simulink library "motohawk_engine_motoshare_lib"  (Simulink 6.3)
undefined symbols (not defined in the file or in its folder): cast_val, IndPowerMax, lookup_group, motohawk_tex, motohawk_vardec_config_group, motohawk_vardec_path, SampleTime, SteadyStateECT, txtTitle, WarmUpTimeConst
libraries: MotoHawk_lib x211, motohawk_control_primitives_lib x20, motohawk_annotations_lib x7, motohawk_engine_lib x5, AutoDoc_lib x4, motohawk_control_primitives_lib_new x3, motohawk_control_primitives_motoshare_lib x2
(part 5 of 7)

== system motohawk_engine_motoshare_lib/PWM Characterization ==
  note: The outputs of this block are designed to be
      | directly connected to a MotoHawk PWM block.
  EngUnits : Inport
  Convert to integer 0.01Hz resolution : Gain  Gain=100  SaturateOnIntegerOverflow=on
  Convert to integer 14-bit PWM resolution : Gain  Gain=40.95  SaturateOnIntegerOverflow=on
  Data Type Conversion1 : DataTypeConversion  SaturateOnIntegerOverflow=on  RndMeth=Zero
  Data Type Conversion2 : DataTypeConversion  OutDataTypeMode=uint32  SaturateOnIntegerOverflow=on  RndMeth=Zero
  Data Type Conversion3 : DataTypeConversion  OutDataTypeMode=int16  SaturateOnIntegerOverflow=on  RndMeth=Zero
  Product : Product  SaturateOnIntegerOverflow=on  InputSameDT=on
  Saturation : motohawk_control_primitives_lib/Saturation
  Sum : Sum  Inputs=|++  SaturateOnIntegerOverflow=on
  motohawk_calibration : MotoHawk_lib/Calibration & Probing Blocks/motohawk_calibration  nam=[prefix 'Gain']  val=1  storage=Calibration  show_more=on  name_source=Use Parameter  data_type=double  read_level=1  write_level=1  ovr_cals=on  view_as=Number  enum_struct={'Disabled', 'Enabled'}  vector_style=Wide Row  use_help_units=on  help='Scaling from engineering units to PWM duty cycle'  units=['%/' units]  use_header_enum=off  row_header_enum={}  col_header_enum={}  use_min_max=off  min_val=-inf  max_val=inf  use_precision=off  precision=''  gain=1  offset=0  exp=1  use_mototune_group=on  mototune_group=[group ' | ' nam ' Config']
  motohawk_calibration1 : MotoHawk_lib/Calibration & Probing Blocks/motohawk_calibration  nam=[prefix 'Offset']  val=0  storage=Calibration  show_more=on  name_source=Use Parameter  data_type=double  read_level=1  write_level=1  ovr_cals=on  view_as=Number  enum_struct={'Disabled', 'Enabled'}  vector_style=Wide Row  use_help_units=on  help='Offset from engineering units to PWM duty cycle'  units='%'  use_header_enum=off  row_header_enum={}  col_header_enum={}  use_min_max=off  min_val=-inf  max_val=inf  use_precision=off  precision=''  gain=1  offset=0  exp=1  use_mototune_group=on  mototune_group=[group ' | ' nam ' Config']
  motohawk_calibration2 : MotoHawk_lib/Calibration & Probing Blocks/motohawk_calibration  nam=[prefix 'MinLimit']  val=0  storage=Calibration  show_more=on  name_source=Use Parameter  data_type=double  read_level=1  write_level=1  ovr_cals=on  view_as=Number  enum_struct={'Disabled', 'Enabled'}  vector_style=Wide Row  use_help_units=on  help='Minimum limit of PWM signal.'  units='%'  use_header_enum=off  row_header_enum={}  col_header_enum={}  use_min_max=off  min_val=-inf  max_val=inf  use_precision=off  precision=''  gain=1  offset=0  exp=1  use_mototune_group=on  mototune_group=[group ' | ' nam ' Config']
  motohawk_calibration3 : MotoHawk_lib/Calibration & Probing Blocks/motohawk_calibration  nam=[prefix 'MaxLimit']  val=100  storage=Calibration  show_more=on  name_source=Use Parameter  data_type=double  read_level=1  write_level=1  ovr_cals=on  view_as=Number  enum_struct={'Disabled', 'Enabled'}  vector_style=Wide Row  use_help_units=on  help='Maximum limit of PWM signal.'  units='%'  use_header_enum=off  row_header_enum={}  col_header_enum={}  use_min_max=off  min_val=-inf  max_val=inf  use_precision=off  precision=''  gain=1  offset=0  exp=1  use_mototune_group=on  mototune_group=[group ' | ' nam ' Config']
  motohawk_calibration4 : MotoHawk_lib/Calibration & Probing Blocks/motohawk_calibration  nam=[prefix 'Frequency']  val=100  storage=Calibration  show_more=on  name_source=Use Parameter  data_type=double  read_level=1  write_level=1  ovr_cals=on  view_as=Number  enum_struct={'Disabled', 'Enabled'}  vector_style=Wide Row  use_help_units=on  help='Frequency of PWM output'  units='Hz'  use_header_enum=off  row_header_enum={}  col_header_enum={}  use_min_max=off  min_val=-inf  max_val=inf  use_precision=off  precision=''  gain=1  offset=0  exp=1  use_mototune_group=on  mototune_group=[group ' | ' nam ' Config']
  motohawk_override_abs2 : MotoHawk_lib/Calibration & Probing Blocks/motohawk_override_abs  parent_name=nam  show_more=on  name_source=Use Parameter  parent_read_level=1  parent_override_level=1  view_as=Number  enum_struct={'Disabled', 'Enabled'}  use_help_units=on  parent_help='Override result of linear sensor characterization, in engineering units'  parent_units=units  use_min_max=on  parent_min=-inf  parent_max=inf  use_precision=off  parent_precision=''  parent_gain=1  parent_offset=0  parent_exp=1  use_mototune_group=on  parent_group=group
  motohawk_probe2 : MotoHawk_lib/Calibration & Probing Blocks/motohawk_probe  nam=[prefix 'DutyCycle']  show_more=on  name_source=Use Parameter  read_level=1  view_as=Number  enum_struct={'Disabled', 'Enabled'}  vector_style=Wide Row  use_help_units=on  help='Actual duty cycle of actuator'  units='%'  use_header_enum=off  row_header_enum={}  col_header_enum={}  use_precision=off  precision=''  gain=1  offset=0  exp=1  use_mototune_group=on  mototune_group=group
  DutyCycle : Outport
  Frequency : Outport  Port=2
  wires:
  Data Type Conversion2/1 -> Frequency/1
  Convert to integer 0.01Hz resolution/1 -> Data Type Conversion2/1
  motohawk_calibration4/1 -> Convert to integer 0.01Hz resolution/1
  Data Type Conversion1/1 -> Product/1
  motohawk_override_abs2/1 -> Data Type Conversion1/1
  EngUnits/1 -> motohawk_override_abs2/1
  Product/1 -> Sum/1
  motohawk_calibration1/1 -> Sum/2
  motohawk_calibration/1 -> Product/2
  Data Type Conversion3/1 -> DutyCycle/1
  Convert to integer 14-bit PWM resolution/1 -> Data Type Conversion3/1
  Sum/1 -> Saturation/1
  Saturation/1 -> Convert to integer 14-bit PWM resolution/1, motohawk_probe2/1
  motohawk_calibration2/1 -> Saturation/2
  motohawk_calibration3/1 -> Saturation/3

== system motohawk_engine_motoshare_lib/Spark Coil Characterization ==
  SparkEnergy [mJ] : Inport
  SysVolt09Idx : Inport  Port=2
  Constant : Constant  Value=1000
  Constant1 : Constant  Value=0
  Only Enable Spark when Energy is Above Zero : RelationalOperator  Operator=>  ZeroCross=off  InputSameDT=on
  Product : Product  Inputs=*/  SaturateOnIntegerOverflow=on
  Sum : Sum  Inputs=|++  SaturateOnIntegerOverflow=on
  motohawk_calibration : MotoHawk_lib/Calibration & Probing Blocks/motohawk_calibration  nam='CoilDrvrDlyTime'  val=0  storage=Calibration  show_more=on  name_source=Use Parameter  data_type=Inherit from 'Default Value'  read_level=1  write_level=1  ovr_cals=on  view_as=Number  enum_struct={'Disabled', 'Enabled'}  vector_style=Wide Row  use_help_units=on  help='Spark Coil Driver Delay Time'  units='us'  use_header_enum=off  row_header_enum={}  col_header_enum={}  use_min_max=off  min_val=-inf  max_val=inf  use_precision=off  precision=''  gain=1  offset=0  exp=1  use_mototune_group=on  mototune_group=[group ' | Coil Config']
  motohawk_interpolation_2d : MotoHawk_lib/Lookup Tables/motohawk_interpolation_2d  nam='CoilDwell'  table_data=ones(9)  show_more=on  data_type=Inherit from 'Table Data'  storage=NonAdaptive  read_level=1  write_level=1  ovr_cals=on  use_help=on  help='Spark dwell time'  units='ms'  use_min_max=off  min_val=-inf  max_val=inf  use_precision=off  precision=''  gain=1  offset=0  exp=1  use_links=on  row_prelookup_block=''  col_prelookup_block=''  output_name='CoilDwell'  use_mototune_group=on  mototune_group=group
  motohawk_prelookup1 : MotoHawk_lib/Lookup Tables/motohawk_prelookup  nam='SpkEnergy09'  breakpoint_data=ones(1,9)  show_more=on  data_type=Inherit from 'Table Data'  storage=Constant  read_level=1  write_level=1  ovr_cals=on  use_help=on  help='Prelookup for Spark Energy'  units='mJ'  use_min_max=off  min_val=-inf  max_val=inf  use_precision=off  precision=''  gain=1  offset=0  exp=1  use_links=on  input_name='SparkEnergy'  use_mototune_group=on  mototune_group='Indexes'
  motohawk_probe : MotoHawk_lib/Calibration & Probing Blocks/motohawk_probe  nam='CoilDwell'  show_more=on  name_source=Use Parameter  read_level=1  view_as=Number  enum_struct={'Disabled', 'Enabled'}  vector_style=Wide Row  use_help_units=on  help='Total electrical spark dwell time'  units='ms'  use_header_enum=off  row_header_enum={}  col_header_enum={}  use_precision=off  precision=''  gain=1  offset=0  exp=1  use_mototune_group=on  mototune_group=group
  motohawk_probe1 : MotoHawk_lib/Calibration & Probing Blocks/motohawk_probe  nam='SparkEnergy'  show_more=on  name_source=Use Parameter  read_level=1  view_as=Number  enum_struct={'Disabled', 'Enabled'}  vector_style=Wide Row  use_help_units=on  help='Commanded spark energy, before conversion to dwell time'  units='mJ'  use_header_enum=off  row_header_enum={}  col_header_enum={}  use_precision=off  precision=''  gain=1  offset=0  exp=1  use_mototune_group=on  mototune_group=group
  SparkDwell [ms] : Outport
  SparkEnable [bool] : Outport  Port=2
  wires:
  Constant1/1 -> Only Enable Spark when Energy is Above Zero/2
  Only Enable Spark when Energy is Above Zero/1 -> SparkEnable [bool]/1
  Constant/1 -> Product/2
  Product/1 -> Sum/2
  motohawk_calibration/1 -> Product/1
  motohawk_interpolation_2d/1 -> Sum/1
  Sum/1 -> SparkDwell [ms]/1, motohawk_probe/1
  SparkEnergy [mJ]/1 -> Only Enable Spark when Energy is Above Zero/1, motohawk_probe1/1, motohawk_prelookup1/1
  motohawk_prelookup1/1 -> motohawk_interpolation_2d/1  "SpkEnergy10Idx"
  SysVolt09Idx/1 -> motohawk_interpolation_2d/2  "SysVolt10Idx"

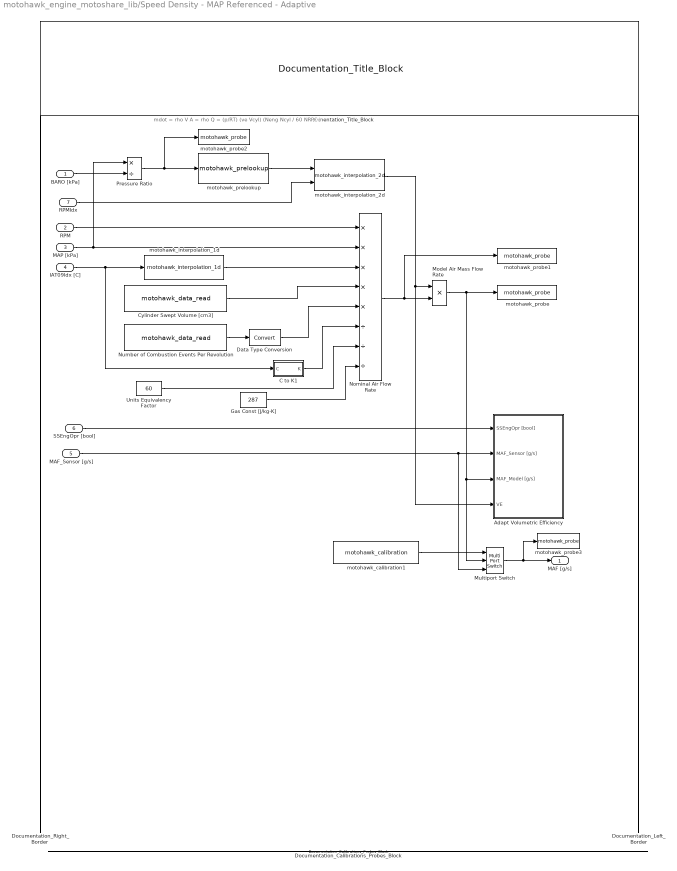
== system motohawk_engine_motoshare_lib/Speed Density - MAP Referenced - Adaptive ==
  note: mdot = rho V A = rho Q = (p/RT) (ve Vcyl) (Neng Ncyl / 60 NRPC )
  BARO [kPa] : Inport
  RPM : Inport  Port=2
  MAP [kPa] : Inport  Port=3
  IAT09Idx [C] : Inport  Port=4
  MAF_Sensor [g/s] : Inport  Port=5
  SSEngOpr [bool] : Inport  Port=6
  RPMIdx : Inport  Port=7
  Adapt Volumetric Efficiency : Subsystem
  C to K1 : Subsystem
      mask Display: disp('to')
  Cylinder Swept Volume [cm3] : MotoHawk_lib/Data Storage Blocks/motohawk_data_read  source=Lookup By Name  structure=Scalar  operation=Read scalar from location by index  sz_vec=-1  sz_row=-1  sz_col=-1  typ=double  nam='CylSweptVol'  checkNull=on  struct_inst_name='Struct1'
  Data Type Conversion : DataTypeConversion  SaturateOnIntegerOverflow=on  RndMeth=Zero
  Documentation_Calibrations_Probes_Block : AutoDoc_lib/Documentation_Calibrations_Probes_Block  pretty_print=off  doc_option=Calibrations and probes display  disp_option=Show border
  Documentation_Left_Border : AutoDoc_lib/Documentation_Left_Border
  Documentation_Right_Border : AutoDoc_lib/Documentation_Right_Border
  Documentation_Title_Block : AutoDoc_lib/Documentation_Title_Block  doc_option=Library block: include in documentation appendix  pretty_print=on  order=1  objcheck=off  obj='Write objectives and requirements here.'  desccheck=on  desc='Write description here.'  eqncheck=on  eqn='Write equations here.'
  Gas Const [J/kg-K] : Constant  Value=287
  Model Air Mass Flow Rate : Product  Inputs=**  SaturateOnIntegerOverflow=on  InputSameDT=on
  Multiport Switch : MultiPortSwitch  Inputs=2  zeroidx=on  SaturateOnIntegerOverflow=on  InputSameDT=on
  Nominal Air Flow Rate : Product  Inputs=*****///  SaturateOnIntegerOverflow=on  InputSameDT=on
  Number of Combustion Events Per Revolution : MotoHawk_lib/Data Storage Blocks/motohawk_data_read  source=Lookup By Name  structure=Scalar  operation=Read scalar from location by index  sz_vec=-1  sz_row=-1  sz_col=-1  typ=uint8  nam='CombEventsPerRev'  checkNull=on  struct_inst_name='Struct1'
  Pressure Ratio : Product  Inputs=*/  SaturateOnIntegerOverflow=on  InputSameDT=on
  Units Equivalency Factor : Constant  Value=60
  motohawk_calibration1 : MotoHawk_lib/Calibration & Probing Blocks/motohawk_calibration  nam='MAF_Source'  val=0  storage=Display  show_more=on  name_source=Use Parameter  data_type=uint8  read_level=1  write_level=1  ovr_cals=on  view_as=Enumeration  enum_struct={'Model from MAP', 'Use MAF sensor directly'}  vector_style=Wide Row  use_help_units=on  help='Selects the source for the fueling algorithm'  units=''  use_header_enum=off  row_header_enum={}  col_header_enum={}  use_min_max=off  min_val=-inf  max_val=inf  use_precision=off  precision=''  gain=1  offset=0  exp=1  use_mototune_group=on  mototune_group=lookup_group(gcb)
  motohawk_interpolation_1d : MotoHawk_lib/Lookup Tables/motohawk_interpolation_1d  nam='VETempCorr'  table_data=ones(1,9)  show_more=on  data_type=Inherit from 'Table Data'  storage=NonAdaptive  read_level=1  write_level=1  ovr_cals=on  use_help=on  help=''  units=''  use_min_max=off  min_val=-inf  max_val=inf  use_precision=off  precision=''  gain=1  offset=0  exp=1  use_links=off  prelookup_block=''  output_name=''  use_mototune_group=on  mototune_group=lookup_group(gcb)
  motohawk_interpolation_2d : MotoHawk_lib/Lookup Tables/motohawk_interpolation_2d  nam='VolEff'  table_data=VolEffMap  show_more=on  data_type=Inherit from 'Table Data'  storage=Adaptive - NonVolatile  read_level=1  write_level=1  ovr_cals=on  use_help=off  help='Volumetric Efficiency'  units='mult'  use_min_max=off  min_val=-inf  max_val=inf  use_precision=off  precision='5.3'  gain=1  offset=0  exp=1  use_links=off  row_prelookup_block=''  col_prelookup_block=''  output_name=''  use_mototune_group=off  mototune_group=lookup_group(gcb)
  motohawk_prelookup : MotoHawk_lib/Lookup Tables/motohawk_prelookup  nam='PressRatio17'  breakpoint_data=PressRatio17IdxArr  show_more=on  data_type=Inherit from 'Table Data'  storage=Constant  read_level=1  write_level=1  ovr_cals=on  use_help=on  help='Prelookup for Pressure Ratio'  units='ratio'  use_min_max=off  min_val=-inf  max_val=inf  use_precision=off  precision=''  gain=1  offset=0  exp=1  use_links=on  input_name='PressRatio'  use_mototune_group=on  mototune_group='Indexes'
  motohawk_probe : MotoHawk_lib/Calibration & Probing Blocks/motohawk_probe  nam='MAF_Model'  show_more=on  name_source=Use Parameter  read_level=1  view_as=Number  enum_struct={'Disabled', 'Enabled'}  vector_style=Wide Row  use_help_units=on  help='Air Mass Flow Rate - Port Total'  units='g/s'  use_header_enum=off  row_header_enum={}  col_header_enum={}  use_precision=off  precision=''  gain=1  offset=0  exp=1  use_mototune_group=on  mototune_group=lookup_group(gcb)
  motohawk_probe1 : MotoHawk_lib/Calibration & Probing Blocks/motohawk_probe  nam='MAF_Ideal'  show_more=on  name_source=Use Parameter  read_level=1  view_as=Number  enum_struct={'Disabled', 'Enabled'}  vector_style=Wide Row  use_help_units=on  help='Air Mass Flow Rate - ideal'  units='g/s'  use_header_enum=off  row_header_enum={}  col_header_enum={}  use_precision=off  precision=''  gain=1  offset=0  exp=1  use_mototune_group=on  mototune_group=lookup_group(gcb)
  motohawk_probe2 : MotoHawk_lib/Calibration & Probing Blocks/motohawk_probe  nam='PressRatio'  show_more=on  name_source=Use Parameter  read_level=1  view_as=Number  enum_struct={'Disabled', 'Enabled'}  vector_style=Wide Row  use_help_units=on  help='Pressure ratio - MAP over BARO'  units='ratio'  use_header_enum=off  row_header_enum={}  col_header_enum={}  use_precision=off  precision=''  gain=1  offset=0  exp=1  use_mototune_group=on  mototune_group=lookup_group(gcb)
  motohawk_probe3 : MotoHawk_lib/Calibration & Probing Blocks/motohawk_probe  nam='MAF'  show_more=on  name_source=Use Parameter  read_level=1  view_as=Number  enum_struct={'Disabled', 'Enabled'}  vector_style=Wide Row  use_help_units=on  help='Air mass flow rate at the intake manifold - Used by the fueling algorithm'  units='g/s'  use_header_enum=off  row_header_enum={}  col_header_enum={}  use_precision=off  precision=''  gain=1  offset=0  exp=1  use_mototune_group=on  mototune_group=lookup_group(gcb)
  MAF [g/s] : Outport
  wires:
  SSEngOpr [bool]/1 -> Adapt Volumetric Efficiency/1(SSEngOpr [bool])
  motohawk_calibration1/1 -> Multiport Switch/1
  Multiport Switch/1 -> motohawk_probe3/1, MAF [g/s]/1
  MAF_Sensor [g/s]/1 -> Adapt Volumetric Efficiency/2(MAF_Sensor [g/s]), Multiport Switch/3
  RPMIdx/1 -> motohawk_interpolation_2d/2
  motohawk_prelookup/1 -> motohawk_interpolation_2d/1
  motohawk_interpolation_2d/1 -> Model Air Mass Flow Rate/1, Adapt Volumetric Efficiency/4(VE)
  Model Air Mass Flow Rate/1 -> Adapt Volumetric Efficiency/3(MAF_Model [g/s]), Multiport Switch/2, motohawk_probe/1
  Pressure Ratio/1 -> motohawk_prelookup/1, motohawk_probe2/1
  IAT09Idx [C]/1 -> C to K1/1(C), motohawk_interpolation_1d/1
  RPM/1 -> Nominal Air Flow Rate/1
  BARO [kPa]/1 -> Pressure Ratio/2
  MAP [kPa]/1 -> Pressure Ratio/1, Nominal Air Flow Rate/2
  Number of Combustion Events Per Revolution/1 -> Data Type Conversion/1
  Nominal Air Flow Rate/1 -> Model Air Mass Flow Rate/2, motohawk_probe1/1
  motohawk_interpolation_1d/1 -> Nominal Air Flow Rate/3
  Cylinder Swept Volume [cm3]/1 -> Nominal Air Flow Rate/4
  Data Type Conversion/1 -> Nominal Air Flow Rate/5
  C to K1/1(K) -> Nominal Air Flow Rate/6
  Units Equivalency Factor/1 -> Nominal Air Flow Rate/7
  Gas Const [J/kg-K]/1 -> Nominal Air Flow Rate/8

== system motohawk_engine_motoshare_lib/Stop Angle to Start Angle ==
  Stop Angle [degCA] : Inport
  RPM : Inport  Port=2
  Duration [ms] : Inport  Port=3
  Product1 : Product  Inputs=**/  SaturateOnIntegerOverflow=on  InputSameDT=on
  Product2 : Product  Inputs=**  SaturateOnIntegerOverflow=on  InputSameDT=on
  Sum : Sum  Inputs=|++  SaturateOnIntegerOverflow=on  InputSameDT=on
  deg/rev : Constant  Value=360
  min/msec : Constant  Value=60000
  Start Angle [degCA] : Outport
  wires:
  Product2/1 -> Sum/2  "PulseWidth [degCA]"
  Product1/1 -> Product2/1  "deg/ms"
  Duration [ms]/1 -> Product2/2  "PulseWidth [ms]"
  deg/rev/1 -> Product1/2
  min/msec/1 -> Product1/3
  RPM/1 -> Product1/1
  Sum/1 -> Start Angle [degCA]/1
  Stop Angle [degCA]/1 -> Sum/1

== system motohawk_engine_motoshare_lib/Capture or Update Signal/Collect Average ==
  note: Collect samples by summing,
      | and divide by the total, to obtain average
  Count : Inport
  Signal : Inport  Port=2
  Enable : EnablePort
  Data Type Conversion : DataTypeConversion  SaturateOnIntegerOverflow=on  RndMeth=Zero
  Product : Product  Inputs=/*
  Sum1 : Sum  Inputs=|++  InputSameDT=on
  Unit Delay1 : UnitDelay  Orientation=left  SampleTime=-1
  Captured_Signal : Outport
  wires:
  Data Type Conversion/1 -> Product/1
  Count/1 -> Data Type Conversion/1
  Product/1 -> Captured_Signal/1
  Signal/1 -> Sum1/1
  Sum1/1 -> Product/2, Unit Delay1/1
  Unit Delay1/1 -> Sum1/2

== system motohawk_engine_motoshare_lib/Crank Synchronous SIgnal/Once at Startup ==
  note: Sample Signal Once at Startup
  Signal_Time : Inport
  f : TriggerPort  TriggerType=function-call
  Signal_StartUp : Outport
  wires:
  Signal_Time/1 -> Signal_StartUp/1

== system motohawk_engine_motoshare_lib/Crank Synchronous SIgnal/TDC and MID_TDC ==
  note: Average of Signal on TDC and MID_TDC
  Signal_Time : Inport
  f : TriggerPort  TriggerType=function-call
  Gain : Gain  Gain=1/2  SaturateOnIntegerOverflow=on
  Sum : Sum  Inputs=|++  InputSameDT=on
  Unit Delay : UnitDelay  SampleTime=-1
  Signal_Ave : Outport
  wires:
  Signal_Time/1 -> Sum/1, Unit Delay/1
  Gain/1 -> Signal_Ave/1
  Sum/1 -> Gain/1
  Unit Delay/1 -> Sum/2

== system motohawk_engine_motoshare_lib/Idle Governor/Idle State Determination ==
  note: Idle States
      | 1 - Flaring
      | 2 - OnIdle
      | 3 - OffIdle
  RPM : Inport
  TargetRPM : Inport  Port=2
  ThrPos [%] : Inport  Port=3
  Determine if RPM is Falling : Subsystem
  Idle State Machine : Stateflow chart
  OnIdle State : motohawk_control_primitives_lib/CompareTo  op===  val=2
  Relational Operator : RelationalOperator  Operator=<  ZeroCross=off  InputSameDT=on
  Relational Operator1 : RelationalOperator  Operator=<  ZeroCross=off  InputSameDT=on
  Relational Operator2 : RelationalOperator  ZeroCross=off  InputSameDT=on
  Sum : Sum  Inputs=|++  SaturateOnIntegerOverflow=on  InputSameDT=on
  motohawk_TitleBlock : motohawk_annotations_lib/motohawk_TitleBlock  BlockType_='Mototron_Title_Block'  ttl='Idle Governor State Determination'  copyright="'THE INFORMATION CONTAINED IN THIS\\newlineDRAWING IS THE SOLE PROPERTY OF\\newlineMOTOTRON.  ANY REPRODUCTION IN\\newline PART OR AS A WHOLE WITHOUT THE\\newlineWRITTEN PERMISSION OF MOTOTRON\\newline IS PROHIBITED.\\fontsize{16}\\rm\\copyright\\rm\\fontsize{10} 2005'"  address='\fontsize{22}\it\fontname{Arial Black}MotoTron Corporation \fontname{Arial}\fontsize{10}\newline505 Marion Road, Oshkosh, WI, 54901\newlinewww.mototron.com (734) 822-7700'  image_file='mh.jpg'  pretty_print=on  edit_text=[motohawk_tex(get_param(bdroot, 'Description')) '\rm\newline' motohawk_tex(get_param(gcs, 'Name'))]  edit_as=6
  motohawk_calibration1 : MotoHawk_lib/Calibration & Probing Blocks/motohawk_calibration  nam='IdleEntryRPMDelta'  val=200  storage=Calibration  show_more=on  name_source=Use Parameter  data_type=Inherit from 'Default Value'  read_level=1  write_level=1  ovr_cals=on  view_as=Number  enum_struct={'Disabled', 'Enabled'}  vector_style=Wide Row  use_help_units=on  help='RPM must be within this delta from IdleTargetRPM to enter the Idle governor'  units='RPM'  use_header_enum=off  row_header_enum={}  col_header_enum={}  use_min_max=off  min_val=-inf  max_val=inf  use_precision=off  precision=''  gain=1  offset=0  exp=1  use_mototune_group=off  mototune_group=motohawk_vardec_path(gcb)
  motohawk_calibration3 : MotoHawk_lib/Calibration & Probing Blocks/motohawk_calibration  nam='IdleEntryThrPosThresh'  val=10  storage=Calibration  show_more=on  name_source=Use Parameter  data_type=Inherit from 'Default Value'  read_level=1  write_level=1  ovr_cals=on  view_as=Number  enum_struct={'Disabled', 'Enabled'}  vector_style=Wide Row  use_help_units=on  help='The throttle position must be closed below this threshold to enter the Idle governor'  units='%'  use_header_enum=off  row_header_enum={}  col_header_enum={}  use_min_max=off  min_val=-inf  max_val=inf  use_precision=off  precision=''  gain=1  offset=0  exp=1  use_mototune_group=off  mototune_group=motohawk_vardec_path(gcb)
  motohawk_calibration4 : MotoHawk_lib/Calibration & Probing Blocks/motohawk_calibration  nam='IdleExitThrPosThresh'  val=15  storage=Calibration  show_more=on  name_source=Use Parameter  data_type=Inherit from 'Default Value'  read_level=1  write_level=1  ovr_cals=on  view_as=Number  enum_struct={'Disabled', 'Enabled'}  vector_style=Wide Row  use_help_units=on  help='The throttle position must be opened above this threshold to exit the Idle governor'  units='%'  use_header_enum=off  row_header_enum={}  col_header_enum={}  use_min_max=off  min_val=-inf  max_val=inf  use_precision=off  precision=''  gain=1  offset=0  exp=1  use_mototune_group=off  mototune_group=motohawk_vardec_path(gcb)
  motohawk_calibration6 : MotoHawk_lib/Calibration & Probing Blocks/motohawk_calibration  nam='IdleEnable'  val=true  storage=Display  show_more=on  name_source=Use Parameter  data_type=Inherit from 'Default Value'  read_level=1  write_level=1  ovr_cals=on  view_as=Number  enum_struct={'Disabled', 'Enabled'}  vector_style=Wide Row  use_help_units=on  help='Allows the Idle governor to be manually enabled and disabled'  units='bool'  use_header_enum=off  row_header_enum={}  col_header_enum={}  use_min_max=off  min_val=-inf  max_val=inf  use_precision=off  precision=''  gain=1  offset=0  exp=1  use_mototune_group=off  mototune_group=motohawk_vardec_path(gcb)
  motohawk_probe1 : MotoHawk_lib/Calibration & Probing Blocks/motohawk_probe  nam='IdleState'  show_more=on  name_source=Use Parameter  read_level=1  view_as=Number  enum_struct={'Disabled', 'Enabled'}  vector_style=Wide Row  use_help_units=on  help="'0 - Off Idle    1 - On Idle'"  units=''  use_header_enum=off  row_header_enum={}  col_header_enum={}  use_precision=off  precision=''  gain=1  offset=0  exp=1  use_mototune_group=off  mototune_group=motohawk_vardec_path(gcb)
  OnIdle : Outport
  wires:
  Relational Operator1/1 -> Idle State Machine/4(ThrPosLow)
  Relational Operator/1 -> Idle State Machine/3(RPMLow)
  OnIdle State/1 -> OnIdle/1
  Idle State Machine/1(IdleState) -> OnIdle State/1, motohawk_probe1/1
  motohawk_calibration6/1 -> Idle State Machine/1(IdleEnable)
  Relational Operator2/1 -> Idle State Machine/5(ThrPosHigh)
  motohawk_calibration4/1 -> Relational Operator2/2
  motohawk_calibration3/1 -> Relational Operator1/2
  Sum/1 -> Relational Operator/2
  motohawk_calibration1/1 -> Sum/1
  TargetRPM/1 -> Sum/2
  Determine if RPM is Falling/1(RPM Falling) -> Idle State Machine/2(RPMFalling)
  RPM/1 -> Determine if RPM is Falling/1(RPM), Relational Operator/1
  ThrPos [%]/1 -> Relational Operator2/1, Relational Operator1/1

== system motohawk_engine_motoshare_lib/Idle Governor/Ramp RPM ==
  note: y[k] = a*x[k] + (1-a)*y[k-1]
  note: where a = t/T
  OnIdle : Inport
  RPM : Inport  Port=2
  TargetRPM : Inport  Port=3
  Constant : Constant
  Logical Operator : Logic  Operator=NOT
  Preload lowpass filter with current RPM while not on Idle : Switch  Threshold=1  ZeroCross=off  SaturateOnIntegerOverflow=on  InputSameDT=on
  Product1 : Product  Inputs=*/  SaturateOnIntegerOverflow=on  InputSameDT=on
  Product2 : Product  SaturateOnIntegerOverflow=on  InputSameDT=on
  Product3 : Product  SaturateOnIntegerOverflow=on  InputSameDT=on
  Sum : Sum  Inputs=-+|  SaturateOnIntegerOverflow=on
  Sum1 : Sum  SaturateOnIntegerOverflow=on
  Unit Delay : UnitDelay  Orientation=left  SampleTime=-1
  motohawk_calibration : MotoHawk_lib/Calibration & Probing Blocks/motohawk_calibration  nam='IdleRPMRampFiltConst'  val=3  storage=Calibration  show_more=on  name_source=Use Parameter  data_type=Inherit from 'Default Value'  read_level=1  write_level=1  ovr_cals=on  view_as=Number  enum_struct={'Disabled', 'Enabled'}  vector_style=Wide Row  use_help_units=on  help='RPM ramp down time constant'  units='sec'  use_header_enum=off  row_header_enum={}  col_header_enum={}  use_min_max=off  min_val=-inf  max_val=inf  use_precision=off  precision=''  gain=1  offset=0  exp=1  use_mototune_group=on  mototune_group=motohawk_vardec_path(gcb)
  motohawk_delta_time : MotoHawk_lib/Extra Development Blocks/motohawk_delta_time  samp_time=SampleTime  init_val=0
  RPMSetPt : Outport
  wires:
  RPM/1 -> Preload lowpass filter with current RPM while not on Idle/1
  TargetRPM/1 -> Product2/1
  Logical Operator/1 -> Preload lowpass filter with current RPM while not on Idle/2
  Product1/1 -> Sum/1, Product2/2  "alpha"
  Constant/1 -> Sum/2
  Product2/1 -> Sum1/1
  Product3/1 -> Sum1/2
  Sum/1 -> Product3/1
  Unit Delay/1 -> Product3/2
  motohawk_delta_time/1 -> Product1/1
  motohawk_calibration/1 -> Product1/2
  Sum1/1 -> Preload lowpass filter with current RPM while not on Idle/3
  Preload lowpass filter with current RPM while not on Idle/1 -> Unit Delay/1, RPMSetPt/1
  OnIdle/1 -> Logical Operator/1

== system motohawk_engine_motoshare_lib/Injector Characterization/FPCOffsets_8Cyl ==
  Fuel In : Inport
  Demux : Demux  Outputs=8
  Mux : Mux  Inputs=8
  motohawk_override_rel : MotoHawk_lib/Calibration & Probing Blocks/motohawk_override_rel  parent_name='Fuel_Cyl1'  show_more=on  name_source=Use Parameter  parent_read_level=1  parent_override_level=1  use_help_units=on  parent_help='Provide lock and relative offset to input signal.'  parent_units='mg'  use_min_max=off  parent_min=-inf  parent_max=inf  use_precision=off  parent_precision=''  parent_gain=1  parent_offset=0  parent_exp=1  use_mototune_group=on  parent_group='Engine Control | Run | Fuel | Liquid'
  motohawk_override_rel1 : MotoHawk_lib/Calibration & Probing Blocks/motohawk_override_rel  parent_name='Fuel_Cyl2'  show_more=on  name_source=Use Parameter  parent_read_level=1  parent_override_level=1  use_help_units=on  parent_help='Provide lock and relative offset to input signal.'  parent_units='mg'  use_min_max=off  parent_min=-inf  parent_max=inf  use_precision=off  parent_precision=''  parent_gain=1  parent_offset=0  parent_exp=1  use_mototune_group=on  parent_group='Engine Control | Run | Fuel | Liquid'
  motohawk_override_rel2 : MotoHawk_lib/Calibration & Probing Blocks/motohawk_override_rel  parent_name='Fuel_Cyl3'  show_more=on  name_source=Use Parameter  parent_read_level=1  parent_override_level=1  use_help_units=on  parent_help='Provide lock and relative offset to input signal.'  parent_units='mg'  use_min_max=off  parent_min=-inf  parent_max=inf  use_precision=off  parent_precision=''  parent_gain=1  parent_offset=0  parent_exp=1  use_mototune_group=on  parent_group='Engine Control | Run | Fuel | Liquid'
  motohawk_override_rel3 : MotoHawk_lib/Calibration & Probing Blocks/motohawk_override_rel  parent_name='Fuel_Cyl4'  show_more=on  name_source=Use Parameter  parent_read_level=1  parent_override_level=1  use_help_units=on  parent_help='Provide lock and relative offset to input signal.'  parent_units='mg'  use_min_max=off  parent_min=-inf  parent_max=inf  use_precision=off  parent_precision=''  parent_gain=1  parent_offset=0  parent_exp=1  use_mototune_group=on  parent_group='Engine Control | Run | Fuel | Liquid'
  motohawk_override_rel4 : MotoHawk_lib/Calibration & Probing Blocks/motohawk_override_rel  parent_name='Fuel_Cyl5'  show_more=on  name_source=Use Parameter  parent_read_level=1  parent_override_level=1  use_help_units=on  parent_help='Provide lock and relative offset to input signal.'  parent_units='mg'  use_min_max=off  parent_min=-inf  parent_max=inf  use_precision=off  parent_precision=''  parent_gain=1  parent_offset=0  parent_exp=1  use_mototune_group=on  parent_group='Engine Control | Run | Fuel | Liquid'
  motohawk_override_rel5 : MotoHawk_lib/Calibration & Probing Blocks/motohawk_override_rel  parent_name='Fuel_Cyl6'  show_more=on  name_source=Use Parameter  parent_read_level=1  parent_override_level=1  use_help_units=on  parent_help='Provide lock and relative offset to input signal.'  parent_units='mg'  use_min_max=off  parent_min=-inf  parent_max=inf  use_precision=off  parent_precision=''  parent_gain=1  parent_offset=0  parent_exp=1  use_mototune_group=on  parent_group='Engine Control | Run | Fuel | Liquid'
  motohawk_override_rel6 : MotoHawk_lib/Calibration & Probing Blocks/motohawk_override_rel  parent_name='Fuel_Global'  show_more=on  name_source=Use Parameter  parent_read_level=1  parent_override_level=1  use_help_units=on  parent_help='Provide lock and relative offset to input signal.'  parent_units='mg'  use_min_max=off  parent_min=-inf  parent_max=inf  use_precision=off  parent_precision=''  parent_gain=1  parent_offset=0  parent_exp=1  use_mototune_group=on  parent_group='Engine Control | Run | Fuel | Liquid'
  motohawk_override_rel7 : MotoHawk_lib/Calibration & Probing Blocks/motohawk_override_rel  parent_name='Fuel_Cyl7'  show_more=on  name_source=Use Parameter  parent_read_level=1  parent_override_level=1  use_help_units=on  parent_help='Provide lock and relative offset to input signal.'  parent_units='mg'  use_min_max=off  parent_min=-inf  parent_max=inf  use_precision=off  parent_precision=''  parent_gain=1  parent_offset=0  parent_exp=1  use_mototune_group=on  parent_group='Engine Control | Run | Fuel | Liquid'
  motohawk_override_rel8 : MotoHawk_lib/Calibration & Probing Blocks/motohawk_override_rel  parent_name='Fuel_Cyl8'  show_more=on  name_source=Use Parameter  parent_read_level=1  parent_override_level=1  use_help_units=on  parent_help='Provide lock and relative offset to input signal.'  parent_units='mg'  use_min_max=off  parent_min=-inf  parent_max=inf  use_precision=off  parent_precision=''  parent_gain=1  parent_offset=0  parent_exp=1  use_mototune_group=on  parent_group='Engine Control | Run | Fuel | Liquid'
  motohawk_probe3 : MotoHawk_lib/Calibration & Probing Blocks/motohawk_probe  nam='TotalFPC'  show_more=on  name_source=Use Parameter  read_level=1  view_as=Number  enum_struct={'Disabled', 'Enabled'}  vector_style=Wide Row  use_help_units=on  help='Total fuel per cylinder after application of transient algorithm'  units='mg'  use_header_enum=off  row_header_enum={}  col_header_enum={}  use_precision=off  precision=''  gain=1  offset=0  exp=1  use_mototune_group=on  mototune_group='Engine Control | Run | Fuel | Liquid'
  Fuel Out : Outport
  wires:
  Demux/1 -> motohawk_override_rel/1
  Demux/2 -> motohawk_override_rel1/1
  Demux/3 -> motohawk_override_rel2/1
  Demux/4 -> motohawk_override_rel3/1
  motohawk_override_rel/1 -> Mux/1
  motohawk_override_rel1/1 -> Mux/2
  motohawk_override_rel2/1 -> Mux/3
  motohawk_override_rel3/1 -> Mux/4
  Fuel In/1 -> Demux/1
  Mux/1 -> motohawk_override_rel6/1
  motohawk_override_rel6/1 -> Fuel Out/1, motohawk_probe3/1
  Demux/5 -> motohawk_override_rel4/1
  motohawk_override_rel4/1 -> Mux/5
  Demux/6 -> motohawk_override_rel5/1
  motohawk_override_rel5/1 -> Mux/6
  Demux/7 -> motohawk_override_rel7/1
  motohawk_override_rel7/1 -> Mux/7
  Demux/8 -> motohawk_override_rel8/1
  motohawk_override_rel8/1 -> Mux/8

== system motohawk_engine_motoshare_lib/Injector Characterization/Fuel dP Arbitration ==
  BARO : Inport
  MAP : Inport  Port=2
  FuelPress : Inport  Port=3
  Const Ref to Atm : Fcn  Expr=u(1) + u(2) - u(3)
  Const Ref to MAP : Fcn  Expr=u(1)
  Multiport Switch : MultiPortSwitch  Inputs=5  zeroidx=on  SaturateOnIntegerOverflow=on
  Mux1 : Mux
  Regulated Gauge Fuel Pressure [kPa]1 : MotoHawk_lib/Calibration & Probing Blocks/motohawk_calibration  nam='InjdPCompType'  val=0  storage=Calibration  show_more=on  name_source=Use Parameter  data_type=int8  read_level=1  write_level=1  ovr_cals=on  view_as=Enumeration  enum_struct={'ConstRefToAtm', 'ConstRefToMAP', 'VariableW/AbsSens', 'VariableW/GaugeSensor' , 'VariableW/GaugeSensorRefToMAP'}  vector_style=Wide Row  use_help_units=on  help='Choose the method of dP calculation, which is used to compensate the fuel pulse width.'  units='option'  use_header_enum=off  row_header_enum={}  col_header_enum={}  use_min_max=off  min_val=-inf  max_val=inf  use_precision=off  precision=''  gain=1  offset=0  exp=1  use_mototune_group=on  mototune_group='Actuators | Injectors | Injector Config'
  Regulated Gauge Fuel Pressure [kPa]2 : MotoHawk_lib/Calibration & Probing Blocks/motohawk_calibration  nam='GaugeFuelPress'  val=343  storage=Calibration  show_more=on  name_source=Use Parameter  data_type=Inherit from 'Default Value'  read_level=1  write_level=1  ovr_cals=on  view_as=Number  enum_struct={'Disabled', 'Enabled'}  vector_style=Wide Row  use_help_units=on  help='Fuel pressure of fuel rail.'  units='kPa'  use_header_enum=off  row_header_enum={}  col_header_enum={}  use_min_max=on  min_val=0  max_val=inf  use_precision=off  precision=''  gain=1  offset=0  exp=1  use_mototune_group=on  mototune_group='Actuators | Injectors | Injector Config'
  Var With Gauge Sensor Ref to Atm : Fcn  Expr=u(4) + u(2) - u(3)
  Var With Gauge Sensor Ref to MAP : Fcn  Expr=u(4)
  Variable with Abs Sensor : Fcn  Expr=u(4)-u(3)
  motohawk_prelookup1 : MotoHawk_lib/Lookup Tables/motohawk_prelookup  nam='InjDeltaPress09'  breakpoint_data=[300 315 325 350 365 385 400 430 450]  show_more=on  data_type=Inherit from 'Table Data'  storage=Constant  read_level=1  write_level=1  ovr_cals=on  use_help=on  help=''  units=''  use_min_max=off  min_val=-inf  max_val=inf  use_precision=on  precision=''  gain=1  offset=0  exp=1  use_links=off  input_name=''  use_mototune_group=on  mototune_group='Indexes'
  motohawk_probe1 : MotoHawk_lib/Calibration & Probing Blocks/motohawk_probe  nam='InjDeltaPress'  show_more=on  name_source=Use Parameter  read_level=1  view_as=Number  enum_struct={'Disabled', 'Enabled'}  vector_style=Wide Row  use_help_units=on  help=''  units=''  use_header_enum=off  row_header_enum={}  col_header_enum={}  use_precision=off  precision=''  gain=1  offset=0  exp=1  use_mototune_group=on  mototune_group='Actuators | Injectors'
  dP : Outport
  DeltaPress09Idx : Outport  Port=2
  wires:
  Regulated Gauge Fuel Pressure [kPa]1/1 -> Multiport Switch/1
  Mux1/1 -> Const Ref to Atm/1, Const Ref to MAP/1, Variable with Abs Sensor/1, Var With Gauge Sensor Ref to Atm/1, Var With Gauge Sensor Ref to MAP/1
  Regulated Gauge Fuel Pressure [kPa]2/1 -> Mux1/1
  BARO/1 -> Mux1/2
  Const Ref to Atm/1 -> Multiport Switch/2
  Multiport Switch/1 -> dP/1, motohawk_probe1/1, motohawk_prelookup1/1
  MAP/1 -> Mux1/3
  FuelPress/1 -> Mux1/4
  Const Ref to MAP/1 -> Multiport Switch/3
  Variable with Abs Sensor/1 -> Multiport Switch/4
  Var With Gauge Sensor Ref to Atm/1 -> Multiport Switch/5
  Var With Gauge Sensor Ref to MAP/1 -> Multiport Switch/6
  motohawk_prelookup1/1 -> DeltaPress09Idx/1

== system motohawk_engine_motoshare_lib/Linear Sensor Characterization/If Action Subsystem ==
  In : Inport
  Action Port : ActionPort
  Out : Outport
  wires:
  In/1 -> Out/1

== system motohawk_engine_motoshare_lib/Linear Sensor Characterization/If Action Subsystem1 ==
  In : Inport
  Action Port : ActionPort
  Out : Outport
  wires:
  In/1 -> Out/1

== system motohawk_engine_motoshare_lib/Linear Sensor Characterization/If Action Subsystem2 ==
  In : Inport
  Action Port : ActionPort
  Out : Outport
  wires:
  In/1 -> Out/1

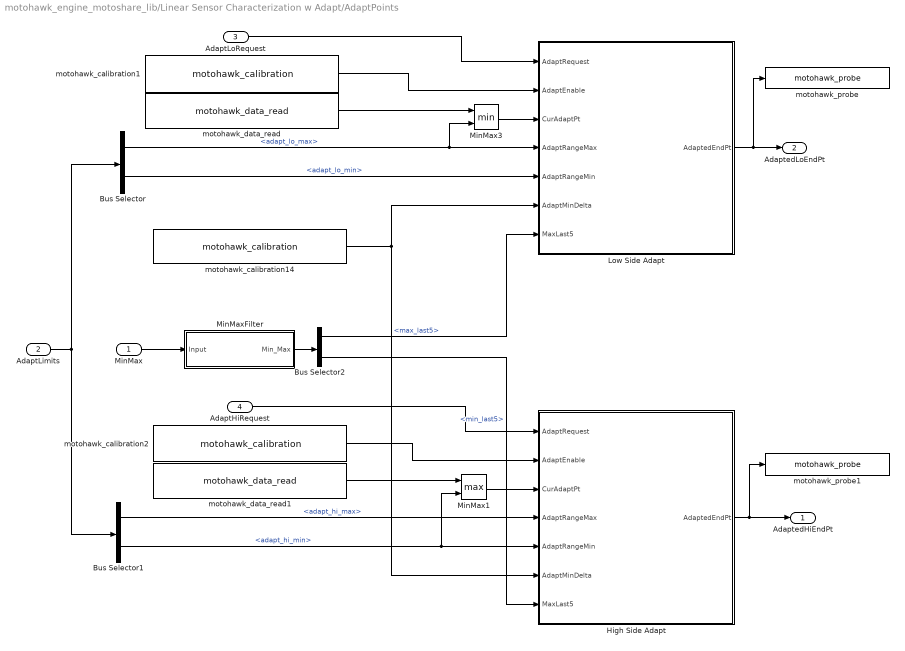
== system motohawk_engine_motoshare_lib/Linear Sensor Characterization w Adapt/AdaptPoints ==
  MinMax : Inport
  AdaptLimits : Inport  Port=2
  AdaptLoRequest : Inport  Port=3
  AdaptHiRequest : Inport  Port=4
  Bus Selector : BusSelector  OutputSignals=adapt_lo_max,adapt_lo_min
  Bus Selector1 : BusSelector  OutputSignals=adapt_hi_max,adapt_hi_min
  Bus Selector2 : BusSelector  OutputSignals=max_last5,min_last5
  High Side Adapt : Subsystem
  Low Side Adapt : Subsystem
  MinMax1 : MinMax  Function=max  Inputs=2
  MinMax3 : MinMax  Inputs=2
  MinMaxFilter : Subsystem
  motohawk_calibration1 : MotoHawk_lib/Calibration & Probing Blocks/motohawk_calibration  nam=[prefix 'AdaptLoEnable']  val=true  storage=Calibration  show_more=on  name_source=Use Parameter  data_type=Inherit from 'Default Value'  read_level=1  write_level=1  ovr_cals=on  view_as=Enumeration  enum_struct={'Disabled', 'Enabled'}  vector_style=Wide Row  use_help_units=on  help='Enables or disables this adapt.'  units=''  use_header_enum=off  row_header_enum={}  col_header_enum={}  use_min_max=off  min_val=-inf  max_val=inf  use_precision=off  precision=''  gain=1  offset=0  exp=1  use_mototune_group=on  mototune_group=[group ' | ' nam ' Config']
  motohawk_calibration14 : MotoHawk_lib/Calibration & Probing Blocks/motohawk_calibration  nam=[prefix 'AdaptDelta']  val=5  storage=Calibration  show_more=on  name_source=Use Parameter  data_type=Inherit from 'Default Value'  read_level=1  write_level=1  ovr_cals=on  view_as=Number  enum_struct={'Disabled', 'Enabled'}  vector_style=Wide Row  use_help_units=on  help='Specifies the minimum deviation amount to react to.'  units='ADC'  use_header_enum=off  row_header_enum={}  col_header_enum={}  use_min_max=off  min_val=-inf  max_val=inf  use_precision=off  precision=''  gain=1  offset=0  exp=1  use_mototune_group=on  mototune_group=[group ' | ' nam ' Config']
  motohawk_calibration2 : MotoHawk_lib/Calibration & Probing Blocks/motohawk_calibration  nam=[prefix 'AdaptHiEnable']  val=true  storage=Calibration  show_more=on  name_source=Use Parameter  data_type=Inherit from 'Default Value'  read_level=1  write_level=1  ovr_cals=on  view_as=Enumeration  enum_struct={'Disabled', 'Enabled'}  vector_style=Wide Row  use_help_units=on  help='Enables or disables this adapt.'  units=''  use_header_enum=off  row_header_enum={}  col_header_enum={}  use_min_max=off  min_val=-inf  max_val=inf  use_precision=off  precision=''  gain=1  offset=0  exp=1  use_mototune_group=on  mototune_group=[group ' | ' nam ' Config']
  motohawk_data_read : MotoHawk_lib/Data Storage Blocks/motohawk_data_read  source=Lookup By Name  structure=Scalar  operation=Read entire data structure at once  sz_vec=4  sz_row=2  sz_col=3  typ=uint16  nam=[prefix 'RawAdptLow']  checkNull=on  struct_inst_name='Struct1'
  motohawk_data_read1 : MotoHawk_lib/Data Storage Blocks/motohawk_data_read  source=Lookup By Name  structure=Scalar  operation=Read entire data structure at once  sz_vec=4  sz_row=2  sz_col=3  typ=uint16  nam=[prefix 'RawAdptHi']  checkNull=on  struct_inst_name='Struct1'
  motohawk_probe : MotoHawk_lib/Calibration & Probing Blocks/motohawk_probe  nam=[prefix 'AdaptLow']  show_more=on  name_source=Use Parameter  read_level=1  view_as=Number  enum_struct={'Disabled', 'Enabled'}  vector_style=Wide Row  use_help_units=on  help=''  units=''  use_header_enum=off  row_header_enum={}  col_header_enum={}  use_precision=on  precision=''  gain=1  offset=0  exp=1  use_mototune_group=on  mototune_group=group
  motohawk_probe1 : MotoHawk_lib/Calibration & Probing Blocks/motohawk_probe  nam=[prefix 'AdaptHi']  show_more=on  name_source=Use Parameter  read_level=1  view_as=Number  enum_struct={'Disabled', 'Enabled'}  vector_style=Wide Row  use_help_units=off  help=''  units=''  use_header_enum=off  row_header_enum={}  col_header_enum={}  use_precision=off  precision=''  gain=1  offset=0  exp=1  use_mototune_group=on  mototune_group=group
  AdaptedHiEndPt : Outport
  AdaptedLoEndPt : Outport  Port=2
  wires:
  MinMaxFilter/1(Min_Max) -> Bus Selector2/1
  Bus Selector2/2 -> High Side Adapt/7(MaxLast5)  "<min_last5>"
  Bus Selector2/1 -> Low Side Adapt/7(MaxLast5)  "<max_last5>"
  MinMax/1 -> MinMaxFilter/1(Input)
  Bus Selector1/2 -> MinMax1/2, High Side Adapt/5(AdaptRangeMin)  "<adapt_hi_min>"
  Bus Selector1/1 -> High Side Adapt/4(AdaptRangeMax)  "<adapt_hi_max>"
  High Side Adapt/1(AdaptedEndPt) -> motohawk_probe1/1, AdaptedHiEndPt/1
  Low Side Adapt/1(AdaptedEndPt) -> motohawk_probe/1, AdaptedLoEndPt/1
  motohawk_calibration14/1 -> Low Side Adapt/6(AdaptMinDelta), High Side Adapt/6(AdaptMinDelta)
  Bus Selector/2 -> Low Side Adapt/5(AdaptRangeMin)  "<adapt_lo_min>"
  Bus Selector/1 -> Low Side Adapt/4(AdaptRangeMax), MinMax3/2  "<adapt_lo_max>"
  AdaptLimits/1 -> Bus Selector1/1, Bus Selector/1
  MinMax3/1 -> Low Side Adapt/3(CurAdaptPt)
  motohawk_data_read/1 -> MinMax3/1
  MinMax1/1 -> High Side Adapt/3(CurAdaptPt)
  motohawk_data_read1/1 -> MinMax1/1
  motohawk_calibration1/1 -> Low Side Adapt/2(AdaptEnable)
  AdaptLoRequest/1 -> Low Side Adapt/1(AdaptRequest)
  motohawk_calibration2/1 -> High Side Adapt/2(AdaptEnable)
  AdaptHiRequest/1 -> High Side Adapt/1(AdaptRequest)

== system motohawk_engine_motoshare_lib/Linear Sensor Characterization w Adapt/Fault Manager Override ==
  Signal : Inport
  Default : Inport  Port=2
  If : If  Orientation=down  NumInputs=2  IfExpression=u1  ElseIfExpressions=u2  ZeroCross=off
  If Action Subsystem : motohawk_engine_lib/Linear Sensor Characterization/If Action Subsystem
  If Action Subsystem1 : motohawk_engine_lib/Linear Sensor Characterization/If Action Subsystem1
  If Action Subsystem2 : motohawk_engine_lib/Linear Sensor Characterization/If Action Subsystem2
  Logical Operator1 : Logic  Operator=OR
  Logical Operator4 : Logic  Operator=OR
  Logical Operator5 : Logic
  Logical Operator6 : Logic  Operator=NOT
  Merge : Merge  Inputs=3
  Override : MotoHawk_lib/Calibration & Probing Blocks/motohawk_override_abs  parent_name=nam  show_more=on  name_source=Use Parameter  parent_read_level=1  parent_override_level=1  view_as=Number  enum_struct={'Disabled', 'Enabled'}  use_help_units=on  parent_help='Override result of linear sensor characterization, in engineering units'  parent_units=units  use_min_max=on  parent_min=-inf  parent_max=inf  use_precision=off  parent_precision=''  parent_gain=1  parent_offset=0  parent_exp=1  use_mototune_group=on  parent_group=group
  Unit Delay1 : UnitDelay  Orientation=left  SampleTime=-1
  motohawk_fault_status1 : MotoHawk_lib/Fault Management Blocks/motohawk_fault_status  source=Lookup By Name  nam=[prefix 'RangeHigh']  status=Active
  motohawk_fault_status2 : MotoHawk_lib/Fault Management Blocks/motohawk_fault_status  source=Lookup By Name  nam=[prefix 'RangeHigh']  status=Suspected
  motohawk_fault_status3 : MotoHawk_lib/Fault Management Blocks/motohawk_fault_status  source=Lookup By Name  nam=[prefix 'RangeLow']  status=Suspected
  motohawk_fault_status4 : MotoHawk_lib/Fault Management Blocks/motohawk_fault_status  source=Lookup By Name  nam=[prefix 'RangeLow']  status=Active
  motohawk_probe2 : MotoHawk_lib/Calibration & Probing Blocks/motohawk_probe  nam=[prefix 'Percent']  show_more=on  name_source=Use Parameter  read_level=1  view_as=Number  enum_struct={'Disabled', 'Enabled'}  vector_style=Wide Row  use_help_units=on  help=''  units=''  use_header_enum=off  row_header_enum={}  col_header_enum={}  use_precision=on  precision=''  gain=1  offset=0  exp=1  use_mototune_group=on  mototune_group=group
  Percent : Outport
  wires:
  Logical Operator4/1 -> If/2, Logical Operator6/1
  Logical Operator1/1 -> Logical Operator5/2
  Logical Operator5/1 -> If/1
  Logical Operator6/1 -> Logical Operator5/1
  motohawk_fault_status4/1 -> Logical Operator4/2
  motohawk_fault_status1/1 -> Logical Operator4/1
  motohawk_fault_status3/1 -> Logical Operator1/2
  motohawk_fault_status2/1 -> Logical Operator1/1
  Override/1 -> motohawk_probe2/1, Percent/1
  Default/1 -> If Action Subsystem1/1
  Unit Delay1/1 -> If Action Subsystem/1
  If/2 -> If Action Subsystem1/Action
  If Action Subsystem1/1 -> Merge/3
  Signal/1 -> If Action Subsystem2/1
  If Action Subsystem/1 -> Merge/2
  If Action Subsystem2/1 -> Merge/1
  If/1 -> If Action Subsystem/Action
  If/3 -> If Action Subsystem2/Action
  Merge/1 -> Unit Delay1/1, Override/1
